simulink model "PV_curve"  (R2024a)
settings: Solver=FixedStepAuto  StartTime=0.0  StopTime=10.0  FixedStep=0.0001  RelTol=1e-3
undefined symbols (not defined in the file or in its folder): National_Instruments, PCI
libraries: cstblocks x3, sldrtlib x2, simulink x1
settings Model: SimulationMode=external  ExtModeTrigDuration=100001  ExtModeArchiveMode=auto  ExtModeArchiveFileName=pv_curve_data  ExtModeArchiveDirName=C:\Users\Eric\nonlinear-adaptive-control-lab-extremum-seeking-photovoltaic-experiment\tugrul-scripts\stored-data\cart-testing\pv-curves  Creator=Eric  LastModifiedBy=Eric
settings HardwareCC: ProdBitPerLong=64  ProdHWDeviceType=Intel->x86-64 (Linux 64)
settings RTWCC: Description=Simulink Desktop Real-Time  SystemTargetFile=sldrt.tlc  TemplateMakefile=sldrt.tmf  TargetLang=C++  RTWCompilerOptimization=on
settings CodeAppCC: MaxIdLength=95
settings SimulinkDesktopRealTimeCC: TargetLibSuffix=_sldrt.a  TargetPreCompLibLocation=C:\Program Files\MATLAB\R2024a\toolbox\sldrt\lib\win64  TargetLangStandard=C++11 (ISO)

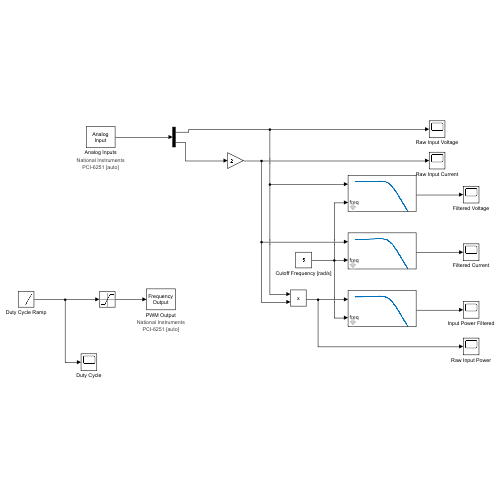
[thumbnail: Simulink's stored preview of the top-level diagram]
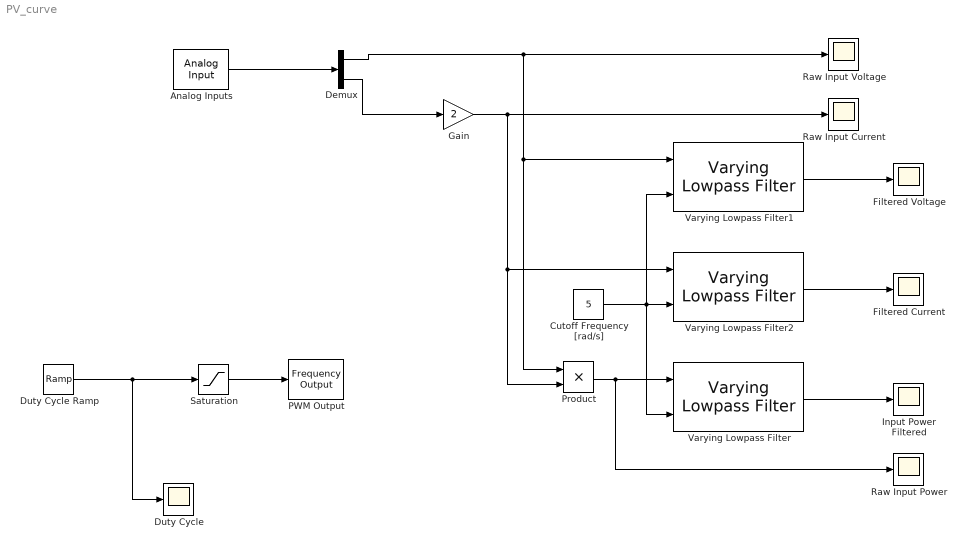
== system PV_curve ==
  Analog Inputs : sldrtlib/Analog Input  SampleTime=0.001  MaxMissedTicks=5000  ShowMissedTicks=off  YieldWhenWaiting=off  DrvName=National_Instruments/PCI-6251  DrvAddress=4294967295  DrvOptions=[1 0 0 3 3]  Channels=[1, 2]  RangeMode=1  VoltRange=1  DataType=1
      settings: AttributesFormatString=National Instruments\nPCI-6251 [auto]
  Cutoff Frequency [rad/s] : Constant  Value=5
  Demux : Demux  Outputs=2
  Duty Cycle : Scope
  Duty Cycle Ramp : simulink/Sources/Ramp  slope=-0.07  start=0  InitialOutput=0.9
  Filtered Current : Scope
  Filtered Voltage : Scope
  Gain : Gain  Gain=2
  Input Power Filtered : Scope
  PWM Output : sldrtlib/Frequency Output  SampleTime=0.0001  MaxMissedTicks=100  ShowMissedTicks=off  YieldWhenWaiting=off  DrvName=National_Instruments/PCI-6251  DrvAddress=4294967295  DrvOptions=[1 0 0 3 3]  Channels=1  FrequencySource=1  Frequency=200000  FrequencyFinalValue=[]  DutySource=2  Duty=[]  DutyFinalValue=[]
      settings: AttributesFormatString=National Instruments\nPCI-6251 [auto]
  Product : Product
  Raw Input Current : Scope
  Raw Input Power : Scope
  Raw Input Voltage : Scope
  Saturation : Saturate  UpperLimit=0.9  LowerLimit=0.2
  Varying Lowpass Filter : cstblocks/Linear Parameter Varying/Varying Lowpass Filter  N=1
  Varying Lowpass Filter1 : cstblocks/Linear Parameter Varying/Varying Lowpass Filter  N=1
  Varying Lowpass Filter2 : cstblocks/Linear Parameter Varying/Varying Lowpass Filter  N=1
  wires:
  Varying Lowpass Filter2/1 -> Filtered Current/1
  Duty Cycle Ramp/1 -> Saturation/1, Duty Cycle/1
  Demux/2 -> Gain/1
  Varying Lowpass Filter1/1 -> Filtered Voltage/1
  Cutoff Frequency [rad/s]/1 -> Varying Lowpass Filter1/2, Varying Lowpass Filter2/2, Varying Lowpass Filter/2
  Product/1 -> Raw Input Power/1, Varying Lowpass Filter/1
  Analog Inputs/1 -> Demux/1
  Demux/1 -> Varying Lowpass Filter1/1, Product/1, Raw Input Voltage/1
  Gain/1 -> Raw Input Current/1, Varying Lowpass Filter2/1, Product/2
  Varying Lowpass Filter/1 -> Input Power Filtered/1
  Saturation/1 -> PWM Output/1
